simulink model "nonlinear_switching_control_closed_loop_system"  (R2020b)
settings: Solver=VariableStepAuto  StartTime=0.0  StopTime=200  RelTol=1e-3
values from neighbouring files (symbols this model uses):
  COMMANDED_TORQUE_SATURATION = 0.05    [Workshop_MATLAB.m]
  COUPLING_COEFFICIENT = 0.5736    [Workshop_MATLAB.m]
  DISTURBANCE_TORQUE = 0.001    [Workshop_MATLAB.m]
  DISTURBANCE_TORQUE_DELAY = 100    [Workshop_MATLAB.m]
  ESTIMATOR_TRANSFER_FUNCTION_DENOMINATOR = [ESTIMATOR_TIME_CONSTANT 1]    [Workshop_MATLAB.m]
  ESTIMATOR_TRANSFER_FUNCTION_NUMERATOR = [1 0]    [Workshop_MATLAB.m]
  FLEXIBLE_MODE_DAMPING_RATIO = 0.00495    [Workshop_MATLAB.m]
  FLEXIBLE_MODE_FREQUENCY = 2.6268    [Workshop_MATLAB.m]
  INITIAL_CONDITION_ON_STATE = 0.0001    [Workshop_MATLAB.m]
  MEASUREMENT_DELAY = 0.8    [Workshop_MATLAB.m]
  MEASUREMENT_NOISE_VARIANCE = 10^(-9)    (= 1e-09)    [Workshop_MATLAB.m]
  modalFeedForwardGain = modalGainMatrixStateFeedback(1)    [Workshop_MATLAB.m]
  modalGainMatrixStateFeedback = [0.517368537052283,6.148270360361254]    [Workshop_MATLAB.m]
  NON_LINEAR_CONTROL_GAIN = 6    [Workshop_MATLAB.m]
  nonLinearControlSpeedCommand = 0.0032    [Workshop_MATLAB.m]
  nonlinearControlswitchingThreshold = nonLinearControlSpeedCommand*modalGainMatrixStateFeedback(2)/modalGainMatrixStateFeedback(1)    [Workshop_MATLAB.m]
  REACTION_WHEEL_DYNAMICS_DENOMINATOR = [1 2.400 0.763]    [Workshop_MATLAB.m]
  REACTION_WHEEL_DYNAMICS_NUMERATOR = REACTION_WHEEL_INERTIA*[1.214 0.763 0]    [Workshop_MATLAB.m]
  REACTION_WHEEL_INERTIA = 0.0004    [Workshop_MATLAB.m]
  REACTION_WHEEL_VELOCITY_SATURATION = 2800*2*pi/60    (= 293.215314335)    [Workshop_MATLAB.m]
  referenceAngle = 0    [Workshop_MATLAB.m]
  SATELLITE_INERTIA = 31.38    [Workshop_MATLAB.m]
  STAR_TRACKER_NOISE_DELAY = 160    [Workshop_MATLAB.m]
libraries: simulink x1
settings Model: Creator=WLCG  LastModifiedBy=WLCG

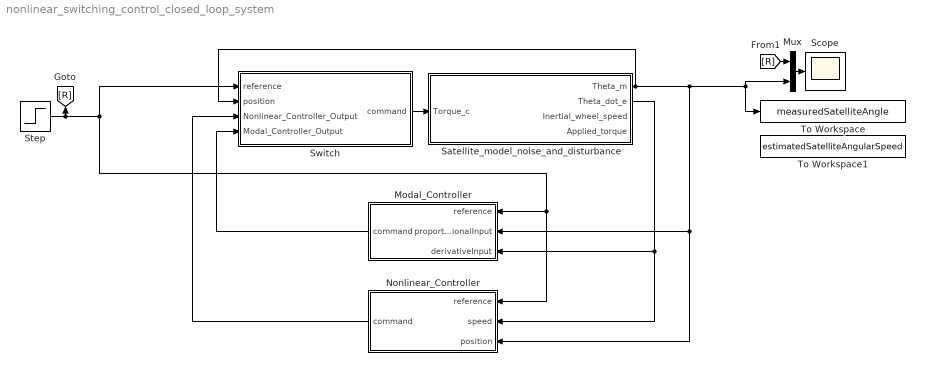
== system nonlinear_switching_control_closed_loop_system ==
  Modal_Controller : Subsystem
  Mux : Mux  Inputs=2
  Nonlinear_Controller : Subsystem
  Satellite_model_noise_and_disturbance : Subsystem
  Scope : Scope
  Step : Step  Time=0  After=referenceAngle  SampleTime=0
  Switch : Subsystem
  To Workspace : ToWorkspace  VariableName=measuredSatelliteAngle  SaveFormat=Timeseries  SampleTime=-1
  To Workspace1 : ToWorkspace  VariableName=estimatedSatelliteAngularSpeed  SaveFormat=Timeseries  SampleTime=-1
  wires:
  Step/1 -> Switch/1(reference), Nonlinear_Controller/1(reference), Modal_Controller/1(reference), [R]
  Satellite_model_noise_and_disturbance/1(Theta_m) -> Modal_Controller/2(proportionalInput), Nonlinear_Controller/3(position), Mux/2, To Workspace/1, Switch/2(position)
  Mux/1 -> Scope/1
  Nonlinear_Controller/1(command) -> Switch/3(Nonlinear_Controller_Output)
  Modal_Controller/1(command) -> Switch/4(Modal_Controller_Output)
  Switch/1(command) -> Satellite_model_noise_and_disturbance/1(Torque_c)
  [R] -> Mux/1
  Satellite_model_noise_and_disturbance/2(Theta_dot_e) -> Modal_Controller/3(derivativeInput), Nonlinear_Controller/2(speed)

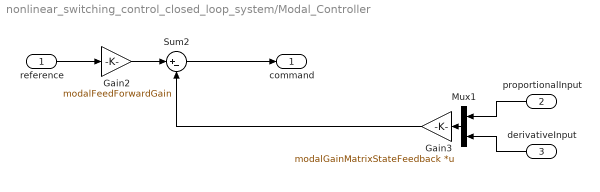
== system nonlinear_switching_control_closed_loop_system/Modal_Controller ==
  reference : Inport
  proportionalInput : Inport  Port=2
  derivativeInput : Inport  Port=3
  Gain2 : Gain  Gain=modalFeedForwardGain
  Gain3 : Gain  Gain=modalGainMatrixStateFeedback  Multiplication=Matrix(K*u)
  Mux1 : Mux  Inputs=2
  Sum2 : Sum  Inputs=|+-
  command : Outport
  wires:
  Mux1/1 -> Gain3/1
  Gain3/1 -> Sum2/2
  Gain2/1 -> Sum2/1
  derivativeInput/1 -> Mux1/2
  Sum2/1 -> command/1
  reference/1 -> Gain2/1
  proportionalInput/1 -> Mux1/1

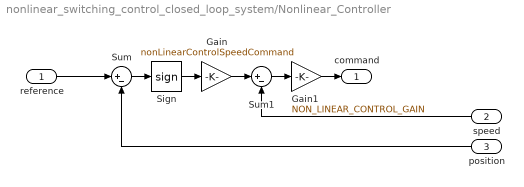
== system nonlinear_switching_control_closed_loop_system/Nonlinear_Controller ==
  reference : Inport
  speed : Inport  Port=2
  position : Inport  Port=3
  Gain : Gain  Gain=nonLinearControlSpeedCommand
  Gain1 : Gain  Gain=NON_LINEAR_CONTROL_GAIN
  Sign : Signum
  Sum : Sum  Inputs=|+-
  Sum1 : Sum  Inputs=|+-
  command : Outport
  wires:
  reference/1 -> Sum/1
  Sum/1 -> Sign/1
  position/1 -> Sum/2
  Sign/1 -> Gain/1
  speed/1 -> Sum1/2
  Gain/1 -> Sum1/1
  Sum1/1 -> Gain1/1
  Gain1/1 -> command/1

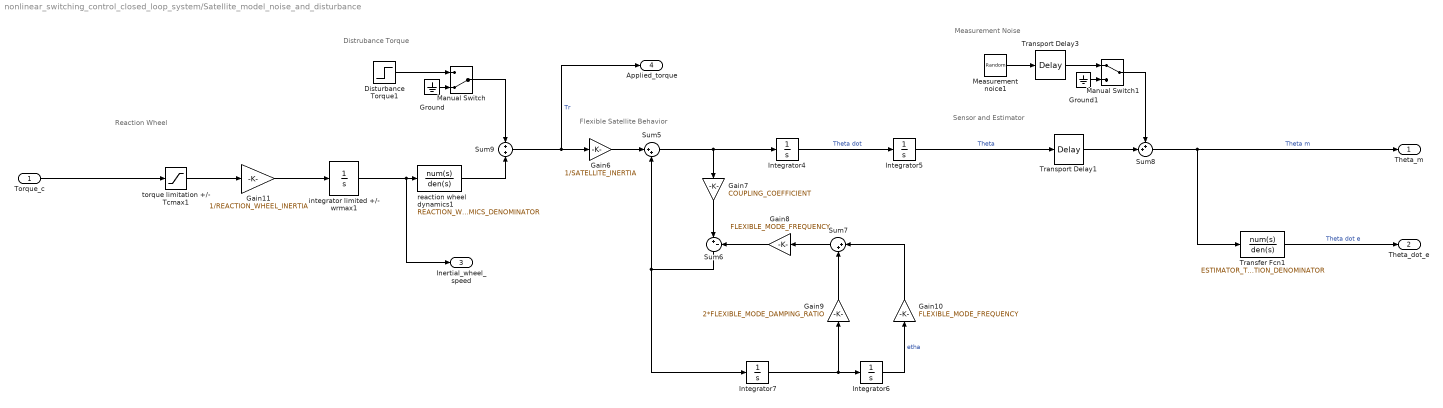
== system nonlinear_switching_control_closed_loop_system/Satellite_model_noise_and_disturbance ==
  note: Distrubance Torque
  note: Measurement Noise
  note: Sensor and Estimator
  note: Flexible Satellite Behavior
  note: Reaction Wheel
  Torque_c : Inport
  Disturbance Torque1 : Step  Time=DISTURBANCE_TORQUE_DELAY  After=DISTURBANCE_TORQUE  SampleTime=0
  Gain10 : Gain  Gain=FLEXIBLE_MODE_FREQUENCY
  Gain11 : Gain  Gain=1/REACTION_WHEEL_INERTIA
  Gain6 : Gain  Gain=1/SATELLITE_INERTIA
  Gain7 : Gain  Gain=COUPLING_COEFFICIENT
  Gain8 : Gain  Gain=FLEXIBLE_MODE_FREQUENCY
  Gain9 : Gain  Gain=2*FLEXIBLE_MODE_DAMPING_RATIO
  Ground : Ground
  Ground1 : Ground
  Integrator4 : Integrator
  Integrator5 : Integrator
  Integrator6 : Integrator  InitialCondition=INITIAL_CONDITION_ON_STATE
  Integrator7 : Integrator
  Manual Switch : ManualSwitch  CurrentSetting=0
  Manual Switch1 : ManualSwitch
  Measurement noice1 : RandomNumber  Variance=MEASUREMENT_NOISE_VARIANCE  SampleTime=0.01
  Sum5 : Sum  Inputs=|++
  Sum6 : Sum  Inputs=|+-
  Sum7 : Sum  Inputs=|++
  Sum8 : Sum  Inputs=++|
  Sum9 : Sum  Inputs=+|+
  Transfer Fcn1 : TransferFcn  Numerator=ESTIMATOR_TRANSFER_FUNCTION_NUMERATOR  Denominator=ESTIMATOR_TRANSFER_FUNCTION_DENOMINATOR
  Transport Delay1 : TransportDelay  DelayTime=MEASUREMENT_DELAY
  Transport Delay3 : TransportDelay  DelayTime=STAR_TRACKER_NOISE_DELAY
  integrator limited +/- wrmax1 : Integrator  LimitOutput=on  UpperSaturationLimit=REACTION_WHEEL_VELOCITY_SATURATION  LowerSaturationLimit=-REACTION_WHEEL_VELOCITY_SATURATION
  reaction wheel dynamics1 : TransferFcn  Numerator=REACTION_WHEEL_DYNAMICS_NUMERATOR  Denominator=REACTION_WHEEL_DYNAMICS_DENOMINATOR
  torque limitation +/- Tcmax1 : Saturate  UpperLimit=COMMANDED_TORQUE_SATURATION  LowerLimit=-COMMANDED_TORQUE_SATURATION
  Theta_m : Outport
  Theta_dot_e : Outport  Port=2
  Inertial_wheel_speed : Outport  Port=3
  Applied_torque : Outport  Port=4
  wires:
  Disturbance Torque1/1 -> Manual Switch/1
  Gain6/1 -> Sum5/1
  Measurement noice1/1 -> Transport Delay3/1
  Gain9/1 -> Sum7/2
  Sum5/1 -> Gain7/1, Integrator4/1
  Gain7/1 -> Sum6/1
  torque limitation +/- Tcmax1/1 -> Gain11/1
  Sum8/1 -> Theta_m/1, Transfer Fcn1/1  "Theta m"
  Sum7/1 -> Gain8/1
  Integrator5/1 -> Transport Delay1/1  "Theta"
  Integrator6/1 -> Gain10/1  "etha"
  Torque_c/1 -> torque limitation +/- Tcmax1/1
  Integrator4/1 -> Integrator5/1  "Theta dot"
  Gain8/1 -> Sum6/2
  Integrator7/1 -> Integrator6/1, Gain9/1
  Sum9/1 -> Applied_torque/1, Gain6/1  "Tr"
  Transfer Fcn1/1 -> Theta_dot_e/1  "Theta dot e"
  Sum6/1 -> Sum5/2, Integrator7/1
  reaction wheel dynamics1/1 -> Sum9/2
  Gain11/1 -> integrator limited +/- wrmax1/1
  Gain10/1 -> Sum7/1
  integrator limited +/- wrmax1/1 -> Inertial_wheel_speed/1, reaction wheel dynamics1/1
  Transport Delay1/1 -> Sum8/2
  Ground/1 -> Manual Switch/2
  Manual Switch/1 -> Sum9/1
  Ground1/1 -> Manual Switch1/2
  Manual Switch1/1 -> Sum8/1
  Transport Delay3/1 -> Manual Switch1/1

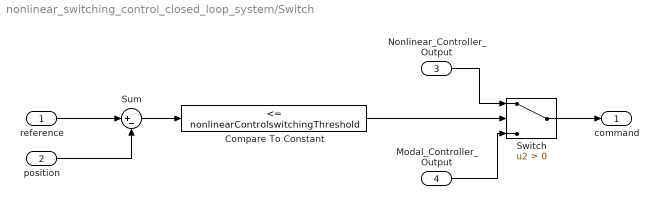
== system nonlinear_switching_control_closed_loop_system/Switch ==
  reference : Inport
  position : Inport  Port=2
  Nonlinear_Controller_Output : Inport  Port=3
  Modal_Controller_Output : Inport  Port=4
  Compare To Constant : simulink/Logic and Bit Operations/Compare To Constant  relop=<=  const=nonlinearControlswitchingThreshold  OutDataTypeStr=boolean
  Sum : Sum  Inputs=|+-
  Switch : Switch  Criteria=u2 > Threshold
  command : Outport
  wires:
  reference/1 -> Sum/1
  Sum/1 -> Compare To Constant/1
  Compare To Constant/1 -> Switch/2
  position/1 -> Sum/2
  Modal_Controller_Output/1 -> Switch/3
  Nonlinear_Controller_Output/1 -> Switch/1
  Switch/1 -> command/1
